simulink model "lab3s"  (R2024b)
settings: Solver=VariableStepAuto  StartTime=0.0  StopTime=10.0  MaxStep=5  RelTol=1e-3
values from neighbouring files (symbols this model uses):
  Cv0 = Pg0    (= 10000)    [lab3.m]
  Cvp = cpp * roo * Vp    (= 75000)    [lab3.m]
  Cvw = cpp * roo * Vw    (= 300000)    [lab3.m]
  czas_skok = 1500    [lab3.m]
  dPg = 0.1 * PgN    (= 1000)    [lab3.m]
  dSP = 10    [lab3.m]
  dTzew = 0    [lab3.m]
  K1 = a * Kp    (= 240)    [lab3.m]
  Kd = (Kp * (TwewN - TpN)) / (TpN - TzewN)    (= 11.4285714286)    [lab3.m]
  Kp = PgN / (a * (TwewN - TzewN) + (TwewN - TpN))    (= 80)    [lab3.m]
  Pg0 = PgN    (= 10000)    [lab3.m]
  RKp = (0.9 * T) / (k * T0)    (= 3085.71428571)    [lab3.m]
  SP0 = Tp0    (= 15)    [lab3.m]
  Ti = 3.33 * T0    (= 832.5)    [lab3.m]
  Tp0 = (Kp / (Kp + Kd)) * (Pg0 / (K1 + (Kp * Kd) / (Kp + Kd))) + Tzew0    (= 15)    [lab3.m]
  Twew0 = (Pg0 / (K1 + (Kp * Kd) / (Kp + Kd))) + Tzew0    (= 20)    [lab3.m]
  Tzew0 = TzewN    (= -20)    [lab3.m]
settings Model: Creator=Adam  LastModifiedBy=Adam

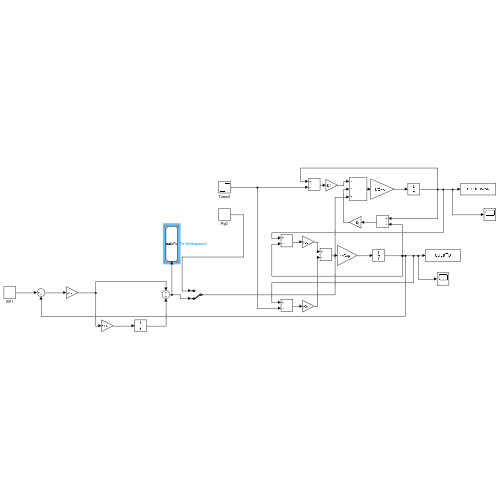
[thumbnail: Simulink's stored preview of the top-level diagram]
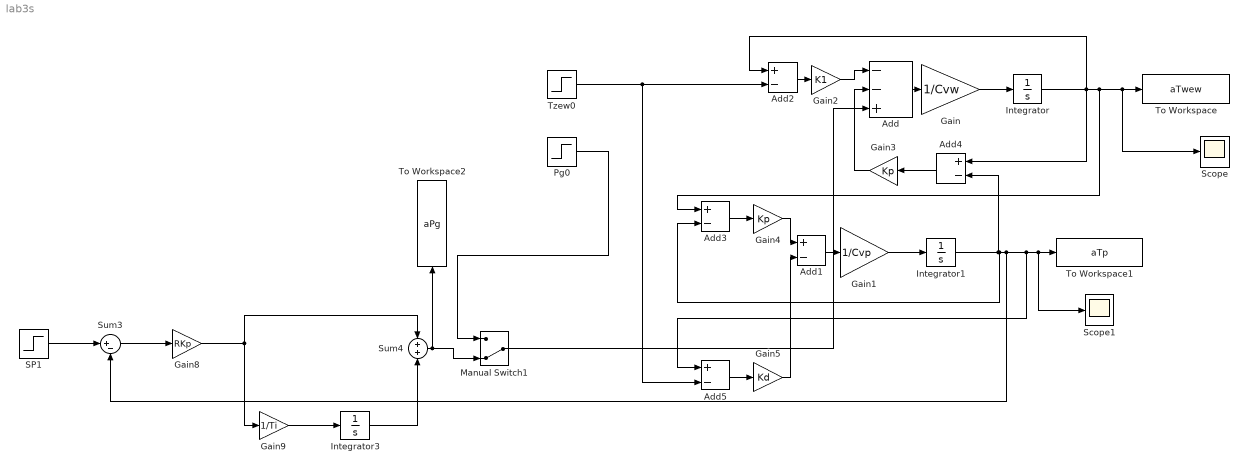
== system lab3s ==
  Add : Sum  Inputs=--+
  Add{1..5} (5 alike) : Sum  Inputs=+-
  Gain : Gain  Gain=1/Cvw
  Gain1 : Gain  Gain=1/Cvp
  Gain2 : Gain  Gain=K1
  Gain3 : Gain  Gain=Kp
  Gain4 : Gain  Gain=Kp
  Gain5 : Gain  Gain=Kd
  Gain8 : Gain  Gain=RKp
  Gain9 : Gain  Gain=1/Ti
  Integrator : Integrator  InitialCondition=Twew0
  Integrator1 : Integrator  InitialCondition=Tp0
  Integrator3 : Integrator  InitialCondition=Cv0
  Manual Switch1 : ManualSwitch  CurrentSetting=0
  Pg0 : Step  Time=czas_skok  Before=Pg0  After=Pg0 + dPg  SampleTime=0
  SP1 : Step  Time=czas_skok  Before=SP0  After=SP0 + dSP  SampleTime=0
  Scope : Scope
  Scope1 : Scope
  Sum3 : Sum  Inputs=|+-
  Sum4 : Sum  Inputs=+|+
  To Workspace : ToWorkspace  VariableName=aTwew  SampleTime=-1
  To Workspace1 : ToWorkspace  VariableName=aTp  SampleTime=-1
  To Workspace2 : ToWorkspace  VariableName=aPg  SampleTime=-1
  Tzew0 : Step  Time=czas_skok  Before=Tzew0  After=Tzew0 + dTzew  SampleTime=0
  wires:
  Add/1 -> Gain/1
  Gain/1 -> Integrator/1
  Add1/1 -> Gain1/1
  Gain1/1 -> Integrator1/1
  Integrator/1 -> Add4/1, Add2/1, Add3/1, Scope/1, To Workspace/1
  Tzew0/1 -> Add5/2, Add2/2
  Add2/1 -> Gain2/1
  Gain2/1 -> Add/1
  Gain3/1 -> Add/2
  Add3/1 -> Gain4/1
  Gain4/1 -> Add1/1
  Add5/1 -> Gain5/1
  Gain5/1 -> Add1/2
  Add4/1 -> Gain3/1
  Pg0/1 -> Manual Switch1/1
  SP1/1 -> Sum3/1
  Integrator3/1 -> Sum4/2
  Gain8/1 -> Gain9/1, Sum4/1
  Sum3/1 -> Gain8/1
  Gain9/1 -> Integrator3/1
  Integrator1/1 -> Add4/2, Add3/2, To Workspace1/1, Scope1/1, Add5/1, Sum3/2
  Sum4/1 -> Manual Switch1/2, To Workspace2/1
  Manual Switch1/1 -> Add/3
